simulink library "nonameslib"  (R2019b)
settings: Solver=VariableStepAuto  StartTime=0.0  StopTime=10.0  RelTol=1e-3
libraries: $bdroot x3
settings Model: Creator=lowlimb  LastModifiedBy=lowlimb

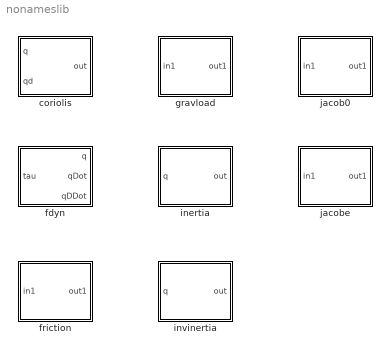
== system nonameslib ==
  coriolis : Subsystem
  fdyn : Subsystem
  friction : MATLAB Function  TreatAsAtomicUnit=on
  gravload : MATLAB Function  TreatAsAtomicUnit=on
  inertia : Subsystem
  invinertia : Subsystem
  jacob0 : MATLAB Function  TreatAsAtomicUnit=on
  jacobe : MATLAB Function  TreatAsAtomicUnit=on

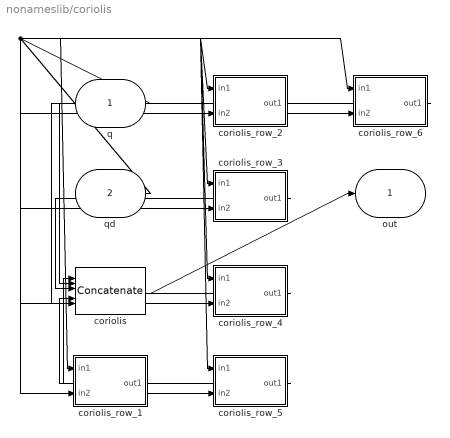
== system nonameslib/coriolis ==
  q : Inport
  qd : Inport  Port=2
  coriolis : Concatenate  NumInputs=6  Mode=Multidimensional array
  coriolis_row_1 : MATLAB Function  TreatAsAtomicUnit=on
  coriolis_row_2 : MATLAB Function  TreatAsAtomicUnit=on
  coriolis_row_3 : MATLAB Function  TreatAsAtomicUnit=on
  coriolis_row_4 : MATLAB Function  TreatAsAtomicUnit=on
  coriolis_row_5 : MATLAB Function  TreatAsAtomicUnit=on
  coriolis_row_6 : MATLAB Function  TreatAsAtomicUnit=on
  out : Outport
  wires:
  coriolis/1 -> out/1
  coriolis_row_1/1(out1) -> coriolis/1
  q/1 -> coriolis_row_1/1(in1), coriolis_row_2/1(in1), coriolis_row_3/1(in1), coriolis_row_4/1(in1), coriolis_row_5/1(in1), coriolis_row_6/1(in1)
  qd/1 -> coriolis_row_1/2(in2), coriolis_row_2/2(in2), coriolis_row_3/2(in2), coriolis_row_4/2(in2), coriolis_row_5/2(in2), coriolis_row_6/2(in2)
  coriolis_row_2/1(out1) -> coriolis/2
  coriolis_row_3/1(out1) -> coriolis/3
  coriolis_row_4/1(out1) -> coriolis/4
  coriolis_row_5/1(out1) -> coriolis/5
  coriolis_row_6/1(out1) -> coriolis/6

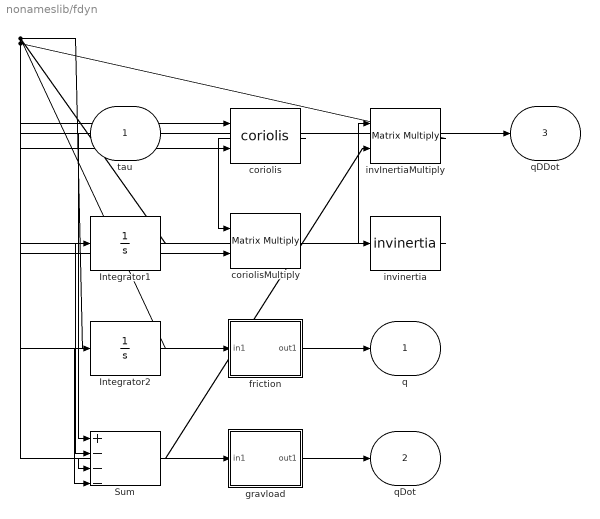
== system nonameslib/fdyn ==
  tau : Inport
  Integrator1 : Integrator
  Integrator2 : Integrator
  Sum : Sum  Inputs=|+---  SaturateOnIntegerOverflow=on  InputSameDT=on  OutDataTypeStr=Inherit: Same as first input
  coriolis : $bdroot/coriolis  SystemSampleTime=-1  Latency=0  AutoFrameSizeCalculation=off
  coriolisMultiply : Product  Multiplication=Matrix(*)  SaturateOnIntegerOverflow=on  RndMeth=Zero  InputSameDT=on  OutDataTypeStr=Inherit: Same as first input
  friction : MATLAB Function  TreatAsAtomicUnit=on
  gravload : MATLAB Function  TreatAsAtomicUnit=on
  invInertiaMultiply : Product  Multiplication=Matrix(*)  SaturateOnIntegerOverflow=on  RndMeth=Zero  InputSameDT=on  OutDataTypeStr=Inherit: Same as first input
  invinertia : $bdroot/invinertia  SystemSampleTime=-1  Latency=0  AutoFrameSizeCalculation=off
  q : Outport
  qDot : Outport  Port=2
  qDDot : Outport  Port=3
  wires:
  tau/1 -> Sum/1
  invInertiaMultiply/1 -> qDDot/1, Integrator1/1
  Integrator1/1 -> Integrator2/1, qDot/1, coriolis/2, coriolisMultiply/2, friction/1(in1)
  Integrator2/1 -> q/1, coriolis/1, gravload/1(in1), invinertia/1
  invinertia/1 -> invInertiaMultiply/1
  Sum/1 -> invInertiaMultiply/2
  coriolisMultiply/1 -> Sum/2
  gravload/1(out1) -> Sum/3
  friction/1(out1) -> Sum/4
  coriolis/1 -> coriolisMultiply/1

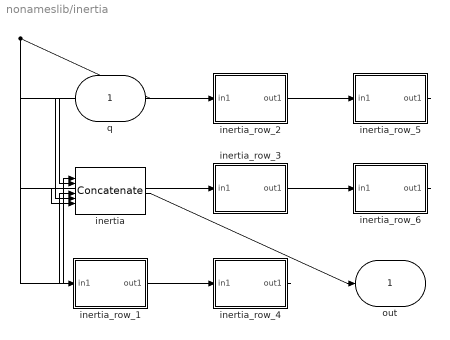
== system nonameslib/inertia ==
  q : Inport
  inertia : Concatenate  NumInputs=6  Mode=Multidimensional array
  inertia_row_1 : MATLAB Function  TreatAsAtomicUnit=on
  inertia_row_2 : MATLAB Function  TreatAsAtomicUnit=on
  inertia_row_3 : MATLAB Function  TreatAsAtomicUnit=on
  inertia_row_4 : MATLAB Function  TreatAsAtomicUnit=on
  inertia_row_5 : MATLAB Function  TreatAsAtomicUnit=on
  inertia_row_6 : MATLAB Function  TreatAsAtomicUnit=on
  out : Outport
  wires:
  inertia/1 -> out/1
  inertia_row_1/1(out1) -> inertia/1
  q/1 -> inertia_row_1/1(in1), inertia_row_2/1(in1), inertia_row_3/1(in1), inertia_row_4/1(in1), inertia_row_5/1(in1), inertia_row_6/1(in1)
  inertia_row_2/1(out1) -> inertia/2
  inertia_row_3/1(out1) -> inertia/3
  inertia_row_4/1(out1) -> inertia/4
  inertia_row_5/1(out1) -> inertia/5
  inertia_row_6/1(out1) -> inertia/6

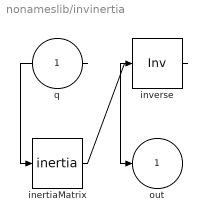
== system nonameslib/invinertia ==
  q : Inport
  inertiaMatrix : $bdroot/inertia  SystemSampleTime=-1  Latency=0  AutoFrameSizeCalculation=off
  inverse : Product  Inputs=/  Multiplication=Matrix(*)
  out : Outport
  wires:
  q/1 -> inertiaMatrix/1
  inertiaMatrix/1 -> inverse/1
  inverse/1 -> out/1

== matlab function nonameslib/inertia/inertia_row_2 ==
  data: in1 input; out1 output
function out1 = inertia_row_2(in1)
%#codegen

%    This function was generated by the Symbolic Math Toolbox version 8.4.
%    03-Apr-2020 15:10:30

q2 = in1(:,2);
q3 = in1(:,3);
q4 = in1(:,4);
q5 = in1(:,5);
t2 = cos(q3);
t3 = cos(q4);
t4 = cos(q5);
t5 = sin(q3);
t6 = sin(q4);
t7 = sin(q5);
t8 = t2.*t3.*(9.0./2.0e+1);
t9 = t2.*t6.*(9.0./2.0e+1);
t10 = t3.*t5.*(9.0./2.0e+1);
t11 = t5.*t6.*(9.0./2.0e+1);
t13 = t2.*t3.*3.3075;
t14 = t2.*t6.*3.3075;
t15 = t3.*t5.*3.3075;
t16 = t5.*t6.*3.3075;
t18 = t2.*2.62458e+1;
t19 = t5.*2.62458e+1;
t20 = t2.*t3.*7.441875e-1;
t21 = t5.*t6.*7.441875e-1;
t23 = t2.*1.181061e+1;
t12 = -t11;
t17 = -t16;
t22 = -t21;
t24 = t9+t10;
t25 = t8+t12+9.0./2.0e+1;
t26 = t4.*t24.*4.326;
t27 = t7.*t24.*4.326;
t29 = t7.*t24.*9.7335e-1;
t28 = -t27;
t30 = -t29;
t31 = t4.*t25.*4.326;
t32 = t7.*t25.*4.326;
t33 = t4.*t25.*9.7335e-1;
t34 = t26+t32;
t38 = t28+t31+9.7335e-1;
t35 = t4.*t34;
t36 = t7.*t34;
t39 = t4.*t38;
t40 = t7.*t38;
t37 = t36.*(9.0./2.0e+1);
t41 = -t40;
t42 = t39.*(9.0./2.0e+1);
t46 = t13+t17+t36+t39+1.65375;
t43 = t14+t15+t35+t41;
t47 = t3.*t46;
t48 = t6.*t46;
t44 = t3.*t43;
t45 = t6.*t43;
t49 = -t48;
t50 = t19+t44+t49;
t52 = t18+t45+t47+2.62458e+1;
t51 = t5.*t50.*(9.0./2.0e+1);
t53 = t2.*t52.*(9.0./2.0e+1);
out1 = [t20+t22+t23+t30+t33+t37+t42+t51+t53+cos(q2).*(t2.*t52+t5.*t50+1.65375).*(9.0./2.0e+1)+sin(q2).*(t2.*t50-t5.*t52).*(9.0./2.0e+1)+1.7031735e+1,t20+t22+t23+t30+t33+t37+t42+t51+t53+1.7031735e+1,t20+t22+t23+t30+t33+t37+t42+1.653561e+1,t20+t22+t30+t33+t37+t42+7.8813e-1,t30+t33+2.92005e-1,0.0];

== matlab function nonameslib/inertia/inertia_row_1 ==
  data: in1 input; out1 output
function out1 = inertia_row_1(in1)
%#codegen

%    This function was generated by the Symbolic Math Toolbox version 8.4.
%    03-Apr-2020 15:10:11

q2 = in1(:,2);
q3 = in1(:,3);
q4 = in1(:,4);
q5 = in1(:,5);
t2 = cos(q2);
t3 = cos(q3);
t4 = cos(q4);
t5 = cos(q5);
t6 = sin(q2);
t7 = sin(q3);
t8 = sin(q4);
t9 = sin(q5);
t10 = t2.*(9.0./2.0e+1);
t11 = t3.*t6.*(9.0./2.0e+1);
t12 = t6.*t7.*(9.0./2.0e+1);
t13 = t2.*7.441875e-1;
t15 = t3.*t6.*2.62458e+1;
t16 = t6.*t7.*2.62458e+1;
t20 = t6.*t7.*1.181061e+1;
t14 = t10+9.0./2.0e+1;
t17 = -t16;
t22 = -t20;
t18 = t3.*t14;
t19 = t7.*t14;
t21 = -t18;
t23 = t18.*5.8324e+1;
t24 = t19.*5.8324e+1;
t25 = t11+t19;
t26 = t18.*2.62458e+1;
t27 = t12+t21;
t28 = t4.*t25;
t29 = t8.*t25;
t30 = t4.*t27;
t31 = t8.*t27;
t33 = t28.*(1.47e+2./2.0e+1);
t34 = t29.*(1.47e+2./2.0e+1);
t38 = t29.*1.65375;
t32 = -t31;
t35 = t30.*(1.47e+2./2.0e+1);
t36 = t31.*(1.47e+2./2.0e+1);
t39 = -t38;
t40 = t30.*1.65375;
t43 = t29+t30-9.0./2.0e+1;
t37 = -t36;
t41 = -t40;
t42 = t28+t32;
t47 = t5.*t43.*4.326;
t48 = t9.*t43.*4.326;
t51 = t5.*t43.*9.7335e-1;
t44 = t5.*t42.*4.326;
t45 = t9.*t42.*4.326;
t46 = t9.*t42.*9.7335e-1;
t50 = -t48;
t52 = -t51;
t49 = -t46;
t53 = t44+t50;
t58 = t45+t47-9.7335e-1;
t54 = t9.*t53;
t55 = t5.*t53;
t59 = t9.*t58;
t60 = t5.*t58;
t56 = -t54;
t57 = t54.*(9.0./2.0e+1);
t61 = t60.*(9.0./2.0e+1);
t63 = t33+t37+t55+t59;
t62 = -t61;
t64 = t4.*t63;
t65 = t8.*t63;
t66 = t34+t35+t56+t60-1.65375;
t67 = t4.*t66;
t68 = t8.*t66;
t69 = -t67;
t70 = t15+t24+t64+t68;
t71 = t7.*t70.*(9.0./2.0e+1);
t72 = t17+t23+t65+t69+2.62458e+1;
t73 = t3.*t72.*(9.0./2.0e+1);
out1 = [t13+t22+t26+t39+t41+t49+t52+t57+t62+t71+t73+t6.*(t6.*3.3075+t3.*t70-t7.*t72).*(9.0./2.0e+1)+t10.*(t2.*3.3075+t3.*t72+t7.*t70+1.65375)+1.732374e+1,t13+t22+t26+t39+t41+t49+t52+t57+t62+t71+t73+1.7031735e+1,t22+t26+t39+t41+t49+t52+t57+t62+1.653561e+1,t39+t41+t49+t52+t57+t62+7.8813e-1,t49+t52+2.92005e-1,0.0];

== matlab function nonameslib/inertia/inertia_row_3 ==
  data: in1 input; out1 output
function out1 = inertia_row_3(in1)
%#codegen

%    This function was generated by the Symbolic Math Toolbox version 8.4.
%    03-Apr-2020 15:10:30

q2 = in1(:,2);
q3 = in1(:,3);
q4 = in1(:,4);
q5 = in1(:,5);
t2 = cos(q3);
t3 = cos(q4);
t4 = cos(q5);
t5 = sin(q3);
t6 = sin(q4);
t7 = sin(q5);
t8 = t7.^2;
t9 = t4.*1.9467;
t11 = t4.*4.380075e-1;
t10 = t7.*t9;
t12 = t8.*1.9467;
t13 = t8.*8.76015e-1;
t14 = t9+9.7335e-1;
t15 = t4.*t14;
t16 = t7.*t14;
t17 = -t16;
t18 = t15.*(9.0./2.0e+1);
t20 = -t3.*(t16-t4.*t7.*1.9467);
t21 = -t6.*(t16-t4.*t7.*1.9467);
t22 = t3.*(t16-t4.*t7.*1.9467);
t23 = t12+t15+1.65375;
t19 = t10+t17;
t24 = t6.*t23;
t25 = t3.*t23;
t26 = t22+t24;
t29 = t21+t25+2.62458e+1;
t27 = t5.*t26.*(9.0./2.0e+1);
t30 = t2.*t29.*(9.0./2.0e+1);
t28 = -t27;
out1 = [t11+t13+t18+t28+t30+cos(q2).*(t2.*t29-t5.*t26).*(9.0./2.0e+1)-sin(q2).*(t2.*t26+t5.*t29).*(9.0./2.0e+1)+1.653561e+1,t11+t13+t18+t28+t30+1.653561e+1,t11+t13+t18+1.653561e+1,t11+t13+t18+7.8813e-1,t11+2.92005e-1,0.0];

== matlab function nonameslib/inertia/inertia_row_4 ==
  data: in1 input; out1 output
function out1 = inertia_row_4(in1)
%#codegen

%    This function was generated by the Symbolic Math Toolbox version 8.4.
%    03-Apr-2020 15:10:31

q2 = in1(:,2);
q3 = in1(:,3);
q4 = in1(:,4);
q5 = in1(:,5);
t2 = cos(q3);
t3 = cos(q4);
t4 = cos(q5);
t5 = sin(q3);
t6 = sin(q4);
t7 = sin(q5);
t8 = t7.^2;
t9 = t4.*1.9467;
t11 = t4.*4.380075e-1;
t10 = t7.*t9;
t12 = t8.*1.9467;
t13 = t8.*8.76015e-1;
t14 = t9+9.7335e-1;
t15 = t4.*t14;
t16 = t7.*t14;
t17 = -t16;
t18 = t15.*(9.0./2.0e+1);
t20 = -t3.*(t16-t4.*t7.*1.9467);
t21 = -t6.*(t16-t4.*t7.*1.9467);
t22 = t3.*(t16-t4.*t7.*1.9467);
t23 = t12+t15+1.65375;
t19 = t10+t17;
t24 = t6.*t23;
t25 = t3.*t23;
t27 = t11+t13+t18+7.8813e-1;
t26 = t21+t25;
t28 = t22+t24;
t29 = t2.*t26.*(9.0./2.0e+1);
t30 = t5.*t28.*(9.0./2.0e+1);
t31 = -t30;
out1 = [t27+t29+t31+cos(q2).*(t2.*t26-t5.*t28).*(9.0./2.0e+1)-sin(q2).*(t2.*t28+t5.*t26).*(9.0./2.0e+1),t27+t29+t31,t27,t27,t11+2.92005e-1,0.0];

== matlab function nonameslib/coriolis/coriolis_row_1 ==
  data: in1 input; out1 output; in2 input
function out1 = coriolis_row_1(in1,in2)
%#codegen

%    This function was generated by the Symbolic Math Toolbox version 8.4.
%    03-Apr-2020 15:11:10

q2 = in1(:,2);
q3 = in1(:,3);
q4 = in1(:,4);
q5 = in1(:,5);
qd1 = in2(:,1);
qd2 = in2(:,2);
qd3 = in2(:,3);
qd4 = in2(:,4);
qd5 = in2(:,5);
t2 = sin(q2);
t3 = sin(q3);
t4 = sin(q5);
t5 = q2+q3;
t6 = q3+q4;
t7 = q4+t5;
t8 = q5+t6;
t9 = sin(t5);
t10 = sin(t6);
t15 = qd2.*t2.*1.49191875e+1;
t17 = qd5.*t4.*4.380075e-1;
t19 = qd3.*t3.*1.181061e+1;
t11 = q5+t7;
t12 = sin(t7);
t13 = sin(t8);
t16 = -t15;
t18 = -t17;
t20 = -t19;
t21 = qd1.*t10.*1.6202025;
t22 = qd2.*t10.*1.6202025;
t23 = qd3.*t10.*1.6202025;
t24 = qd4.*t10.*1.6202025;
t25 = qd1.*t9.*1.181061e+1;
t26 = qd2.*t9.*1.181061e+1;
t27 = qd3.*t9.*1.181061e+1;
t14 = sin(t11);
t28 = qd1.*t13.*4.380075e-1;
t29 = qd2.*t13.*4.380075e-1;
t30 = qd3.*t13.*4.380075e-1;
t31 = qd4.*t13.*4.380075e-1;
t32 = qd5.*t13.*4.380075e-1;
t38 = -t21;
t39 = -t22;
t40 = -t23;
t41 = -t24;
t42 = -t25;
t43 = -t26;
t44 = -t27;
t50 = qd1.*t12.*1.6202025;
t51 = qd2.*t12.*1.6202025;
t52 = qd3.*t12.*1.6202025;
t53 = qd4.*t12.*1.6202025;
t33 = qd1.*t14.*4.380075e-1;
t34 = qd2.*t14.*4.380075e-1;
t35 = qd3.*t14.*4.380075e-1;
t36 = qd4.*t14.*4.380075e-1;
t37 = qd5.*t14.*4.380075e-1;
t45 = -t28;
t46 = -t29;
t47 = -t30;
t48 = -t31;
t49 = -t32;
t59 = -t50;
t60 = -t51;
t61 = -t52;
t62 = -t53;
t54 = -t33;
t55 = -t34;
t56 = -t35;
t57 = -t36;
t58 = -t37;
out1 = [t16+t18+t20+t40+t41+t43+t44+t47+t48+t49+t55+t56+t57+t58+t60+t61+t62,t16+t18+t20+t40+t41+t42+t43+t44+t47+t48+t49+t54+t55+t56+t57+t58+t59+t60+t61+t62-qd1.*t2.*1.49191875e+1,t18+t20+t38+t39+t40+t41+t42+t43+t44+t45+t46+t47+t48+t49+t54+t55+t56+t57+t58+t59+t60+t61+t62-qd1.*t3.*1.181061e+1-qd2.*t3.*1.181061e+1,t18+t38+t39+t40+t41+t45+t46+t47+t48+t49+t54+t55+t56+t57+t58+t59+t60+t61+t62,(t4+t13+t14).*(qd1+qd2+qd3+qd4+qd5).*(-4.380075e-1),0.0];

== matlab function nonameslib/coriolis/coriolis_row_2 ==
  data: in1 input; out1 output; in2 input
function out1 = coriolis_row_2(in1,in2)
%#codegen

%    This function was generated by the Symbolic Math Toolbox version 8.4.
%    03-Apr-2020 15:11:11

q2 = in1(:,2);
q3 = in1(:,3);
q4 = in1(:,4);
q5 = in1(:,5);
qd1 = in2(:,1);
qd2 = in2(:,2);
qd3 = in2(:,3);
qd4 = in2(:,4);
qd5 = in2(:,5);
t2 = sin(q3);
t3 = sin(q5);
t4 = q3+q4;
t5 = q5+t4;
t6 = sin(t4);
t8 = qd5.*t3.*4.380075e-1;
t10 = qd3.*t2.*1.181061e+1;
t7 = sin(t5);
t9 = -t8;
t11 = -t10;
t12 = qd1.*t6.*1.6202025;
t13 = qd2.*t6.*1.6202025;
t14 = qd3.*t6.*1.6202025;
t15 = qd4.*t6.*1.6202025;
t16 = qd1.*t7.*4.380075e-1;
t17 = qd2.*t7.*4.380075e-1;
t18 = qd3.*t7.*4.380075e-1;
t19 = qd4.*t7.*4.380075e-1;
t20 = qd5.*t7.*4.380075e-1;
t21 = -t12;
t22 = -t13;
t23 = -t14;
t24 = -t15;
t25 = -t16;
t26 = -t17;
t27 = -t18;
t28 = -t19;
t29 = -t20;
out1 = [t9+t11+t23+t24+t27+t28+t29+qd1.*sin(q2+q3).*1.181061e+1+qd1.*sin(q2+t4).*1.6202025+qd1.*sin(q2+t5).*4.380075e-1+qd1.*sin(q2).*1.49191875e+1,t9+t11+t23+t24+t27+t28+t29,t9+t11+t21+t22+t23+t24+t25+t26+t27+t28+t29-qd1.*t2.*1.181061e+1-qd2.*t2.*1.181061e+1,t9+t21+t22+t23+t24+t25+t26+t27+t28+t29,(t3+t7).*(qd1+qd2+qd3+qd4+qd5).*(-4.380075e-1),0.0];

== matlab function nonameslib/coriolis/coriolis_row_3 ==
  data: in1 input; out1 output; in2 input
function out1 = coriolis_row_3(in1,in2)
%#codegen

%    This function was generated by the Symbolic Math Toolbox version 8.4.
%    03-Apr-2020 15:11:11

q2 = in1(:,2);
q3 = in1(:,3);
q4 = in1(:,4);
q5 = in1(:,5);
qd1 = in2(:,1);
qd2 = in2(:,2);
qd3 = in2(:,3);
qd4 = in2(:,4);
qd5 = in2(:,5);
t2 = sin(q3);
t3 = sin(q5);
t4 = q3+q4;
t5 = q5+t4;
t6 = sin(t4);
t8 = qd5.*t3.*4.380075e-1;
t10 = qd1.*t2.*1.181061e+1;
t11 = qd2.*t2.*1.181061e+1;
t7 = sin(t5);
t9 = -t8;
t12 = qd1.*t6.*1.6202025;
t13 = qd2.*t6.*1.6202025;
t14 = qd1.*t7.*4.380075e-1;
t15 = qd2.*t7.*4.380075e-1;
out1 = [t9+t10+t11+t12+t13+t14+t15+qd1.*sin(q2+q3).*1.181061e+1+qd1.*sin(q2+t4).*1.6202025+qd1.*sin(q2+t5).*4.380075e-1,t9+t10+t11+t12+t13+t14+t15,t9,t9,t3.*(qd1+qd2+qd3+qd4+qd5).*(-4.380075e-1),0.0];

== matlab function nonameslib/coriolis/coriolis_row_4 ==
  data: in1 input; out1 output; in2 input
function out1 = coriolis_row_4(in1,in2)
%#codegen

%    This function was generated by the Symbolic Math Toolbox version 8.4.
%    03-Apr-2020 15:11:11

q2 = in1(:,2);
q3 = in1(:,3);
q4 = in1(:,4);
q5 = in1(:,5);
qd1 = in2(:,1);
qd2 = in2(:,2);
qd3 = in2(:,3);
qd4 = in2(:,4);
qd5 = in2(:,5);
t2 = sin(q5);
t3 = q3+q4;
t4 = q5+t3;
t5 = sin(t3);
t7 = qd5.*t2.*4.380075e-1;
t6 = sin(t4);
t8 = -t7;
t9 = qd1.*t5.*1.6202025;
t10 = qd2.*t5.*1.6202025;
t11 = qd1.*t6.*4.380075e-1;
t12 = qd2.*t6.*4.380075e-1;
out1 = [t8+t9+t10+t11+t12+qd1.*sin(q2+t3).*1.6202025+qd1.*sin(q2+t4).*4.380075e-1,t8+t9+t10+t11+t12,t8,t8,t2.*(qd1+qd2+qd3+qd4+qd5).*(-4.380075e-1),0.0];

== matlab function nonameslib/gravload ==
  data: in1 input; out1 output
function out1 = gravload(in1)
%#codegen

%    This function was generated by the Symbolic Math Toolbox version 8.4.
%    03-Apr-2020 15:10:35

out1 = [0.0,0.0,0.0,0.0,0.0,0.0];

== matlab function nonameslib/friction ==
  data: in1 input; out1 output
function out1 = friction(in1)
%#codegen

%    This function was generated by the Symbolic Math Toolbox version 8.4.
%    01-Apr-2020 19:54:44

out1 = [0.0,0.0,0.0,0.0];

== matlab function nonameslib/fdyn/gravload ==
  data: in1 input; out1 output
function out1 = gravload(in1)
%#codegen

%    This function was generated by the Symbolic Math Toolbox version 8.4.
%    01-Apr-2020 19:54:42

out1 = [0.0,0.0,0.0,0.0];

== matlab function nonameslib/fdyn/friction ==
  data: in1 input; out1 output
function out1 = friction(in1)
%#codegen

%    This function was generated by the Symbolic Math Toolbox version 8.4.
%    01-Apr-2020 19:54:44

out1 = [0.0,0.0,0.0,0.0];

== matlab function nonameslib/inertia/inertia_row_5 ==
  data: in1 input; out1 output
function out1 = inertia_row_5(in1)
%#codegen

%    This function was generated by the Symbolic Math Toolbox version 8.4.
%    03-Apr-2020 15:10:32

q2 = in1(:,2);
q3 = in1(:,3);
q4 = in1(:,4);
q5 = in1(:,5);
t2 = cos(q3);
t3 = cos(q4);
t4 = cos(q5);
t5 = sin(q3);
t6 = sin(q4);
t7 = sin(q5);
t8 = t3.*t4.*9.7335e-1;
t9 = t3.*t7.*9.7335e-1;
t10 = t4.*t6.*9.7335e-1;
t11 = t6.*t7.*9.7335e-1;
t12 = t4.*4.380075e-1;
t13 = -t11;
t14 = t9+t10;
t19 = t12+2.92005e-1;
t15 = t8+t13;
t16 = t5.*t14.*(9.0./2.0e+1);
t17 = t2.*t15.*(9.0./2.0e+1);
t18 = -t16;
out1 = [t17+t18+t19+cos(q2).*(t2.*t15-t5.*t14).*(9.0./2.0e+1)-sin(q2).*(t2.*t14+t5.*t15).*(9.0./2.0e+1),t17+t18+t19,t19,t19,2.92005e-1,0.0];

== matlab function nonameslib/inertia/inertia_row_6 ==
  data: in1 input; out1 output
function out1 = inertia_row_6(in1)
%#codegen

%    This function was generated by the Symbolic Math Toolbox version 8.4.
%    03-Apr-2020 15:10:32

out1 = [0.0,0.0,0.0,0.0,0.0,0.0];

== matlab function nonameslib/jacob0 ==
  data: in1 input; out1 output
function out1 = jacob0(in1)
%#codegen

%    This function was generated by the Symbolic Math Toolbox version 8.4.
%    03-Apr-2020 15:10:38

q1 = in1(:,1);
q2 = in1(:,2);
q3 = in1(:,3);
q4 = in1(:,4);
q5 = in1(:,5);
q6 = in1(:,6);
t2 = cos(q6);
t3 = sin(q6);
t4 = q5+q6;
t5 = cos(t4);
t6 = sin(t4);
t7 = q3+q4+t4;
t14 = t2.*(9.0./2.0e+1);
t15 = t3.*(9.0./2.0e+1);
t8 = cos(t7);
t9 = q2+t7;
t10 = sin(t7);
t18 = t5.*(9.0./2.0e+1);
t19 = t6.*(9.0./2.0e+1);
t11 = q1+t9;
t12 = sin(t9);
t13 = cos(t9);
t20 = t8.*(9.0./2.0e+1);
t21 = t10.*(9.0./2.0e+1);
t24 = t14+t18;
t25 = t15+t19;
t16 = cos(t11);
t17 = sin(t11);
t22 = t13.*(9.0./2.0e+1);
t23 = t12.*(9.0./2.0e+1);
t31 = t20+t24;
t32 = t21+t25;
t26 = t16.*t24;
t27 = t17.*t24;
t28 = t16.*t25;
t29 = t17.*t25;
t33 = t23+t32;
t34 = t22+t31;
t30 = -t27;
t35 = t26+t29;
t36 = t28+t30;
out1 = reshape([t16.*t33-t17.*t34,t16.*t34+t17.*t33,0.0,0.0,0.0,1.0,t16.*t32-t17.*t31,t16.*t31+t17.*t32,0.0,0.0,0.0,1.0,t36,t35,0.0,0.0,0.0,1.0,t36,t35,0.0,0.0,0.0,1.0,t2.*t17.*(-9.0./2.0e+1)+t15.*t16,t14.*t16+t15.*t17,0.0,0.0,0.0,1.0,0.0,0.0,0.0,0.0,0.0,1.0],[6,6]);

== matlab function nonameslib/jacobe ==
  data: in1 input; out1 output
function out1 = jacobe(in1)
%#codegen

%    This function was generated by the Symbolic Math Toolbox version 8.4.
%    03-Apr-2020 15:10:38

q2 = in1(:,2);
q3 = in1(:,3);
q4 = in1(:,4);
q5 = in1(:,5);
q6 = in1(:,6);
t2 = cos(q6);
t3 = sin(q6);
t4 = q5+q6;
t5 = cos(t4);
t6 = sin(t4);
t7 = q3+q4+t4;
t11 = t2.*(9.0./2.0e+1);
t12 = t3.*(9.0./2.0e+1);
t8 = cos(t7);
t9 = q2+t7;
t10 = sin(t7);
t13 = t5.*(9.0./2.0e+1);
t14 = t6.*(9.0./2.0e+1);
t15 = t8.*(9.0./2.0e+1);
t16 = t10.*(9.0./2.0e+1);
t17 = t11+t13;
t18 = t12+t14;
out1 = reshape([t16+t18+sin(t9).*(9.0./2.0e+1),t15+t17+cos(t9).*(9.0./2.0e+1),0.0,0.0,0.0,1.0,t16+t18,t15+t17,0.0,0.0,0.0,1.0,t18,t17,0.0,0.0,0.0,1.0,t18,t17,0.0,0.0,0.0,1.0,t12,t11,0.0,0.0,0.0,1.0,0.0,0.0,0.0,0.0,0.0,1.0],[6,6]);

== matlab function nonameslib/coriolis/coriolis_row_5 ==
  data: in1 input; out1 output; in2 input
function out1 = coriolis_row_5(in1,in2)
%#codegen

%    This function was generated by the Symbolic Math Toolbox version 8.4.
%    03-Apr-2020 15:11:11

q2 = in1(:,2);
q3 = in1(:,3);
q4 = in1(:,4);
q5 = in1(:,5);
qd1 = in2(:,1);
qd2 = in2(:,2);
qd3 = in2(:,3);
qd4 = in2(:,4);
t2 = sin(q5);
t3 = q3+q4+q5;
t4 = qd1+qd2+qd3+qd4;
t5 = sin(t3);
t6 = qd1.*t2.*4.380075e-1;
t7 = qd2.*t2.*4.380075e-1;
t8 = qd3.*t2.*4.380075e-1;
t9 = qd4.*t2.*4.380075e-1;
t12 = t2.*t4.*4.380075e-1;
t10 = qd1.*t5.*4.380075e-1;
t11 = qd2.*t5.*4.380075e-1;
out1 = [t6+t7+t8+t9+t10+t11+qd1.*sin(q2+t3).*4.380075e-1,t6+t7+t8+t9+t10+t11,t12,t12,0.0,0.0];

== matlab function nonameslib/coriolis/coriolis_row_6 ==
  data: in1 input; out1 output; in2 input
function out1 = coriolis_row_6(in1,in2)
%#codegen

%    This function was generated by the Symbolic Math Toolbox version 8.4.
%    03-Apr-2020 15:11:12

out1 = [0.0,0.0,0.0,0.0,0.0,0.0];
